simulink model "detect_color_hsv"  (R2016b)
settings: Solver=VariableStepAuto  StartTime=0.0  StopTime=10.0  RelTol=1e-3
undefined symbols (not defined in the file or in its folder): Rec, SDTV
libraries: visionconversions x4, visionsources x1
settings Model: Creator=sk  LastModifiedBy=sk

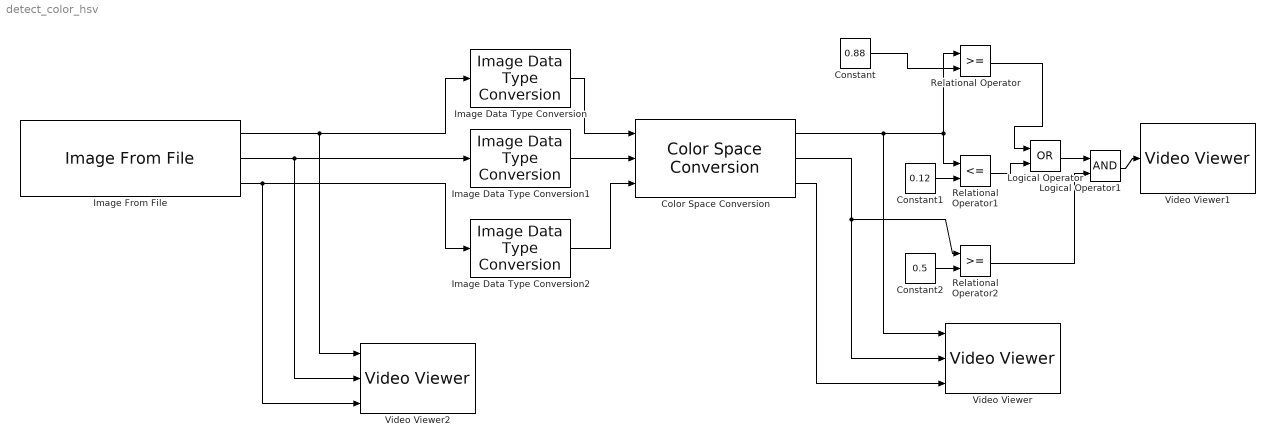
== system detect_color_hsv ==
  Color Space Conversion : visionconversions/Color Space  Conversion  conversion=Obsolete  conversionActive=R'G'B' to HSV  wp_str=D65  rec=Rec. 601 (SDTV)  sys=1125/60/2:1  imagePorts=Separate color signals
  Constant : Constant  Value=0.88
  Constant1 : Constant  Value=0.12
  Constant2 : Constant  Value=0.5
  Image Data Type Conversion : visionconversions/Image Data Type Conversion  outDT=double  isSigned=on  wordLen=16  numFracBits=0
  Image Data Type Conversion1 : visionconversions/Image Data Type Conversion  outDT=double  isSigned=on  wordLen=16  numFracBits=0
  Image Data Type Conversion2 : visionconversions/Image Data Type Conversion  outDT=double  isSigned=on  wordLen=16  numFracBits=0
  Image From File : visionsources/Image From File  Tag=vipblks_nd  FileName=D:\users\skconan\Workspace\MBD\Vision\circle.jpg  imagePorts=Separate color signals  Ts=inf  ImageDataType=Inherit from input image  Signed=on  WordLength=16  sdImageDataType=uint(8)  FractionLengthMode=User-defined  FractionLength=15  OutPortLabels=R|G|B
  Logical Operator : Logic  Operator=OR  AllPortsSameDT=off  OutDataTypeStr=boolean
  Logical Operator1 : Logic  AllPortsSameDT=off  OutDataTypeStr=boolean
  Relational Operator : RelationalOperator  OutDataTypeStr=boolean  RndMeth=Simplest
  Relational Operator1 : RelationalOperator  Operator=<=  OutDataTypeStr=boolean  RndMeth=Simplest
  Relational Operator2 : RelationalOperator  OutDataTypeStr=boolean  RndMeth=Simplest
  Video Viewer : VideoViewer  imagePorts=separate color signals  FigPos=[436 524 410 300]
  Video Viewer1 : VideoViewer  FigPos=[751 534 410 300]
  Video Viewer2 : VideoViewer  imagePorts=separate color signals  FigPos=[53 503 410 300]
  wires:
  Image From File/1 -> Video Viewer2/1, Image Data Type Conversion/1
  Color Space Conversion/1 -> Relational Operator/1, Relational Operator1/1, Video Viewer/1
  Image Data Type Conversion/1 -> Color Space Conversion/1
  Image From File/2 -> Video Viewer2/2, Image Data Type Conversion1/1
  Image From File/3 -> Video Viewer2/3, Image Data Type Conversion2/1
  Image Data Type Conversion1/1 -> Color Space Conversion/2
  Image Data Type Conversion2/1 -> Color Space Conversion/3
  Color Space Conversion/2 -> Relational Operator2/1, Video Viewer/2
  Color Space Conversion/3 -> Video Viewer/3
  Constant/1 -> Relational Operator/2
  Relational Operator/1 -> Logical Operator/1
  Constant1/1 -> Relational Operator1/2
  Relational Operator1/1 -> Logical Operator/2
  Logical Operator/1 -> Logical Operator1/1
  Constant2/1 -> Relational Operator2/2
  Relational Operator2/1 -> Logical Operator1/2
  Logical Operator1/1 -> Video Viewer1/1
